simulink model "sim"  (R2024b)
settings: Solver=VariableStepAuto  StartTime=0.0  StopTime=10.0  RelTol=1e-3
InitFcn:
  | run("main_simulink.mlx");
values from neighbouring files (symbols this model uses):
  i = 1    [dynamicParameters.m]    (also in mpcLoop.m = i+1; mpcLoop_mex.m = i+1; simCooperativeTransport_temp.m = 2)
  x_f = zeros(sys.n, max_iter)    [dynamicParameters.m]
  x_l = zeros(sys.n, max_iter)    [dynamicParameters.m]
settings Model: Creator=kovac  LastModifiedBy=kovac

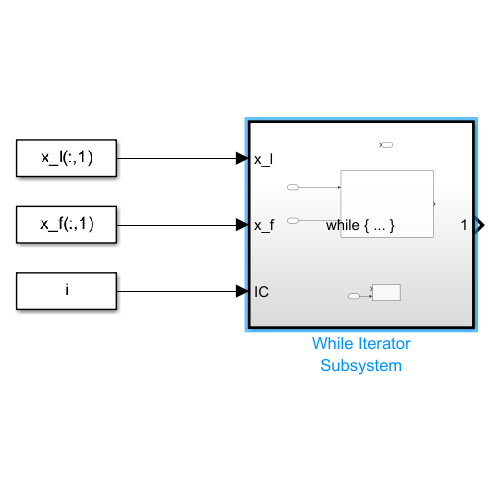
[thumbnail: Simulink's stored preview of the top-level diagram]
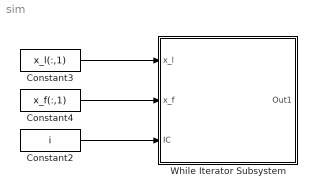
== system sim ==
  Constant2 : Constant  Value=i
  Constant3 : Constant  Value=x_l(:,1)
  Constant4 : Constant  Value=x_f(:,1)
  While Iterator Subsystem : Subsystem  TreatAsAtomicUnit=on
  wires:
  Constant2/1 -> While Iterator Subsystem/3(IC)
  Constant4/1 -> While Iterator Subsystem/2(x_f)
  Constant3/1 -> While Iterator Subsystem/1(x_l)

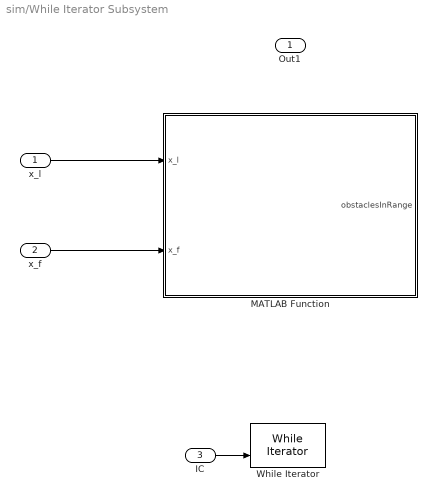
== system sim/While Iterator Subsystem ==
  x_l : Inport
  x_f : Inport  Port=2
  IC : Inport  Port=3
  MATLAB Function : MATLAB Function  TreatAsAtomicUnit=on
  While Iterator : WhileIterator  MaxIters=max_iter
  Out1 : Outport
  wires:
  IC/1 -> While Iterator/2
  x_l/1 -> MATLAB Function/1(x_l)
  x_f/1 -> MATLAB Function/2(x_f)

== matlab function sim/While Iterator Subsystem/MATLAB Function ==
  data: obstaclesInRange output; x_l input; x_f input; obstacles parameter
function obstaclesInRange = evaluateObstacles(x_l, x_f, obstacles)

obstaclesInRange = evaluateObstacles(obstacles, x_l(1:2), x_f(1:2), leaderParams, followerParams, loadParams, sys, N, noise);

if size(obstaclesInRange.qi_l, 1) == 0
    leaderParams.alg = 'active-set';
else
    leaderParams.alg = opt.alg;
end
